simulink model "exnb4137986_Q3"  (R2023b)
settings: Solver=FixedStepAuto  StartTime=0.0  StopTime=20  FixedStep=0.01  RelTol=1e-3
values from neighbouring files (symbols this model uses):
  u_star_1 = double(subs(u_eq, x2, x2_star_1))    [exnb4137986_Q3_par.m]    (also in exnb4137986_Q5_par.m; exnb4137986_Q6_par.m)
  values = [0.005, 10]    [exnb4137986_Q3_par.m]    (also in exnb4137986_Q5_par.m; exnb4137986_Q6_par.m)
  x_star_1 = [x1_star_1, x2_star_1]    [exnb4137986_Q3_par.m]    (also in exnb4137986_Q5_par.m; exnb4137986_Q6_par.m)
settings Model: Creator=therkelsen  LastModifiedBy=therkelsen

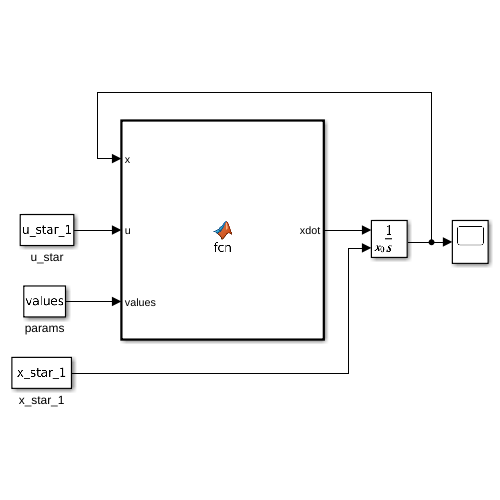
[thumbnail: Simulink's stored preview of the top-level diagram]
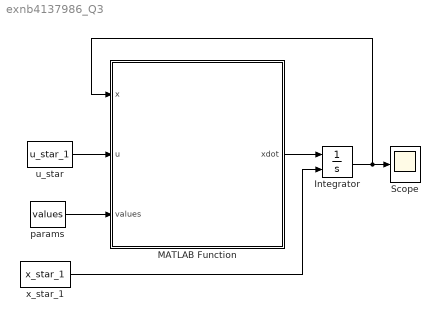
== system exnb4137986_Q3 ==
  Integrator : Integrator  InitialConditionSource=external
  MATLAB Function : MATLAB Function  TreatAsAtomicUnit=on
  Scope : Scope
  params : Constant  Value=values
  u_star : Constant  Value=u_star_1
  x_star_1 : Constant  Value=x_star_1
  wires:
  Integrator/1 -> MATLAB Function/1(x), Scope/1
  x_star_1/1 -> Integrator/2
  MATLAB Function/1(xdot) -> Integrator/1
  params/1 -> MATLAB Function/3(values)
  u_star/1 -> MATLAB Function/2(u)

== matlab function exnb4137986_Q3/MATLAB Function ==
  data: x input; u input; xdot output; values input
function xdot = fcn(x, u, values)

d = values(1);
lambda = values(2);

xdot = [-d*x(1)*abs(x(1)) + x(2);
         -lambda*x(2) + u];
